simulink model "A_2"  (R2021b)
settings: Solver=VariableStepAuto  StartTime=0.0  StopTime=0.3  RelTol=1e-3
model workspace (MAT data in the model file):
  Var = 0
values from neighbouring files (symbols this model uses):
  A1 = [0 0 1 0 ; 0 0 0 1 ; 0 A132 A133 A134 ; 0 A142 A143 A144]    [NXTway_model.m]    (also in SS_matrices.m)
  A2 = [0 1 ; 0 -J/I]    [NXTway_model.m]    (also in SS_matrices.m)
  B1 = [0 0 ; 0 0 ; B13 B13 ; B14 B14]    [NXTway_model.m]    (also in SS_matrices.m)
  B2 = [0 0 ; -K/I K/I]    [NXTway_model.m]    (also in SS_matrices.m)
  C1 = [1 0 0 0 ; 0 1 0 0]    [SS_matrices.m]
  C2 = [1 0]    [SS_matrices.m]
  D1 = [0 0 ; 0 0]    [SS_matrices.m]
  D2 = [0 0]    [SS_matrices.m]
settings Model: Creator=oliverschamp  LastModifiedBy=oliverschamp

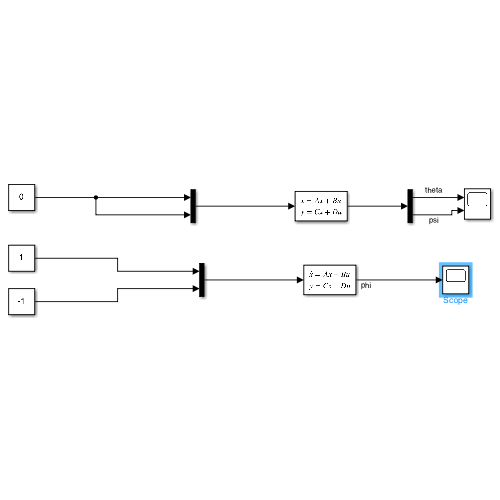
[thumbnail: Simulink's stored preview of the top-level diagram]
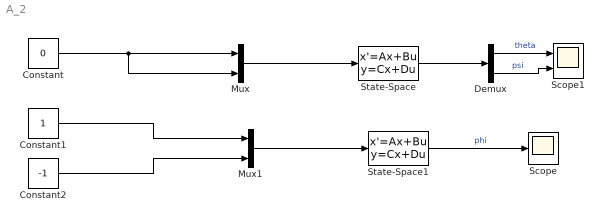
== system A_2 ==
  Constant : Constant  Value=0
  Constant1 : Constant
  Constant2 : Constant  Value=-1
  Demux : Demux  Outputs=2
  Mux : Mux  Inputs=2
  Mux1 : Mux  Inputs=2
  Scope : Scope
  Scope1 : Scope  NumInputPorts=2
  State-Space : StateSpace  A=A1  B=B1  C=C1  D=D1  InitialCondition=[0 20 0 0]  ParameterTunability=Optimized  ContinuousStateAttributes='balance'
  State-Space1 : StateSpace  A=A2  B=B2  C=C2  D=D2  InitialCondition=0
  wires:
  Mux/1 -> State-Space/1
  State-Space/1 -> Demux/1
  Demux/1 -> Scope1/1  "theta"
  Demux/2 -> Scope1/2  "psi"
  Constant/1 -> Mux/2, Mux/1
  Mux1/1 -> State-Space1/1
  State-Space1/1 -> Scope/1  "phi"
  Constant1/1 -> Mux1/1
  Constant2/1 -> Mux1/2
